simulink model "rfpsc"  (R2023b)
settings: Solver=VariableStepAuto  StartTime=0.0  StopTime=.5  RelTol=1e-3
undefined symbols (not defined in the file): f_sw, K_p, L_f, L_g, R_a, R_L, T_s, U_dc, u_gN, w_b, w_g
libraries: simulink x1
settings Model: Creator=maatt  LastModifiedBy=maatt
settings DataIOCC: ReturnWorkspaceOutputs=off

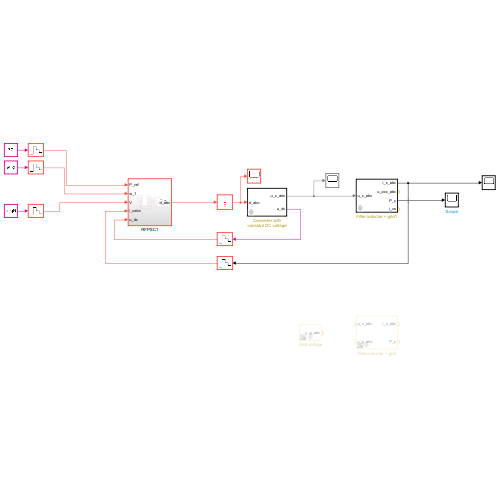
[thumbnail: Simulink's stored preview of the top-level diagram]
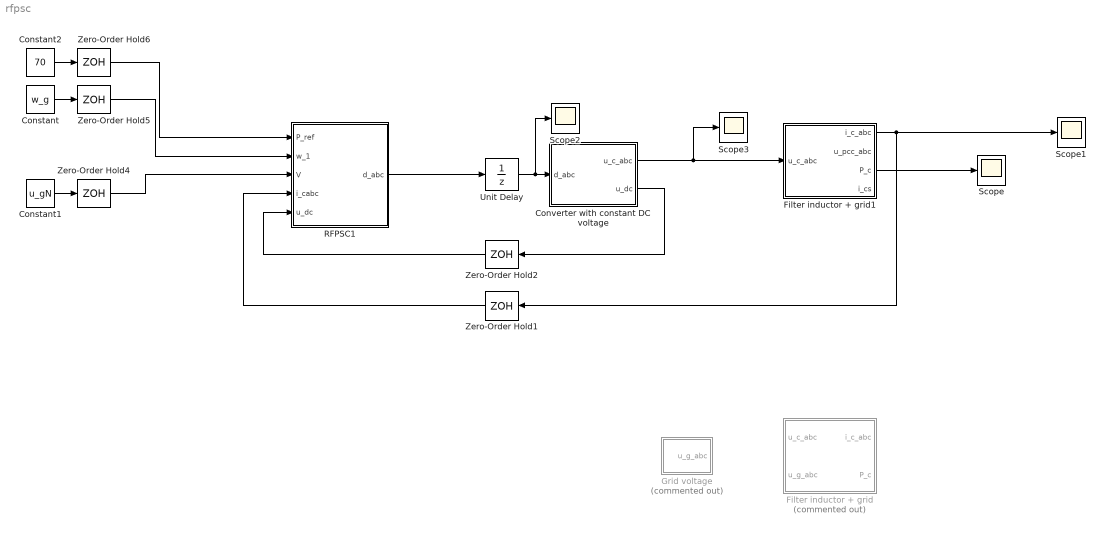
== system rfpsc ==
  Constant : Constant  Value=w_g
  Constant1 : Constant  Value=u_gN
  Constant2 : Constant  Value=70
  "Converter with constant DC voltage " : Subsystem  mask{f_sw=f_sw, u_dc=U_dc}
      mask prompts: f_sw "Switching frequency (Hz)"; u_dc "DC-bus voltage (V)"
      mask init:
      | T_s = 1/(2*f_sw);
  Filter inductor + grid : Subsystem  Commented=on  mask{L_f=L_f, L_g=L_g, R_L=R_L}
      mask prompts: L_f "Filter inductance (H)"; L_g "Grid inductance (H)"; R_L "Series resistance (ohm)"
  Filter inductor + grid1 : Subsystem  mask{L_f=L_f, L_g=L_g, R_L=R_L}
      mask prompts: L_f "Filter inductance (H)"; L_g "Grid inductance (H)"; R_L "Series resistance (ohm)"
  Grid voltage : Subsystem  Commented=on  mask{w_g=2*pi*50, U_g=24}
      mask prompts: w_g "Grid angular frequency (rad/s)"; U_g "Line-to-neutral peak voltage (V)"
  RFPSC1 : Subsystem
  Scope{,1..3} (4 alike) : Scope
  Unit Delay : UnitDelay  SampleTime=T_s  HasFrameUpgradeWarning=on
  Zero-Order Hold{1..2,4..6} (5 alike) : ZeroOrderHold  SampleTime=T_s
  wires:
  "Converter with constant DC voltage "/1(u_c_abc) -> Filter inductor + grid1/1(u_c_abc), Scope3/1
  RFPSC1/1(d_abc) -> Unit Delay/1
  "Converter with constant DC voltage "/2(u_dc) -> Zero-Order Hold2/1
  Constant/1 -> Zero-Order Hold5/1
  Constant1/1 -> Zero-Order Hold4/1
  Unit Delay/1 -> Scope2/1, "Converter with constant DC voltage "/1(d_abc)
  Zero-Order Hold1/1 -> RFPSC1/4(i_cabc)
  Zero-Order Hold4/1 -> RFPSC1/3(V)
  Zero-Order Hold5/1 -> RFPSC1/2(w_1)
  Zero-Order Hold6/1 -> RFPSC1/1(P_ref)
  Zero-Order Hold2/1 -> RFPSC1/5(u_dc)
  Constant2/1 -> Zero-Order Hold6/1
  Filter inductor + grid1/1(i_c_abc) -> Scope1/1, Zero-Order Hold1/1
  Filter inductor + grid1/3(P_c) -> Scope/1

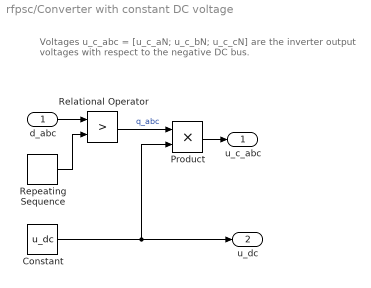
== system rfpsc/Converter with constant DC voltage  ==
  note: Voltages u_c_abc = [u_c_aN; u_c_bN; u_c_cN] are the inverter
      | output voltages with respect to the negative DC bus.
  d_abc : Inport
  Constant : Constant  Value=u_dc
  Product : Product
  Relational Operator : RelationalOperator  Operator=>  OutDataTypeStr='double'  InputSameDT=off
  Repeating Sequence : simulink/Sources/Repeating Sequence  rep_seq_t=[0 1 2]*T_s  rep_seq_y=[1 0 1]
  u_c_abc : Outport
  u_dc : Outport  Port=2
  wires:
  Repeating Sequence/1 -> Relational Operator/2
  d_abc/1 -> Relational Operator/1
  Product/1 -> u_c_abc/1
  Relational Operator/1 -> Product/1  "q_abc"
  Constant/1 -> Product/2, u_dc/1

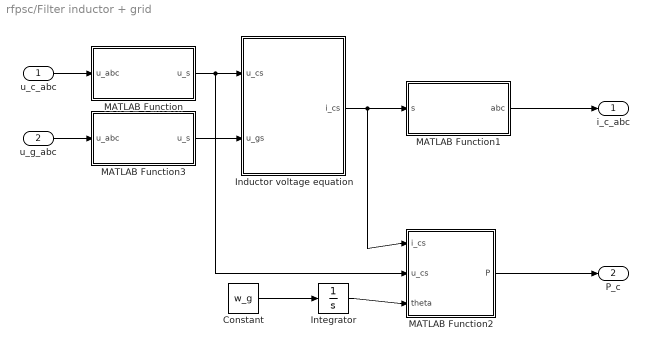
== system rfpsc/Filter inductor + grid ==
  u_c_abc : Inport
  u_g_abc : Inport  Port=2
  Constant : Constant  Value=w_g
  Inductor voltage equation : Subsystem
  Integrator : Integrator  WrapState=on
  MATLAB Function : MATLAB Function  TreatAsAtomicUnit=on
  MATLAB Function1 : MATLAB Function  TreatAsAtomicUnit=on
  MATLAB Function2 : MATLAB Function  TreatAsAtomicUnit=on
  MATLAB Function3 : MATLAB Function  TreatAsAtomicUnit=on
  i_c_abc : Outport
  P_c : Outport  Port=2
  wires:
  u_c_abc/1 -> MATLAB Function/1(u_abc)
  MATLAB Function/1(u_s) -> MATLAB Function2/2(u_cs), Inductor voltage equation/1(u_cs)
  u_g_abc/1 -> MATLAB Function3/1(u_abc)
  MATLAB Function3/1(u_s) -> Inductor voltage equation/2(u_gs)
  Inductor voltage equation/1(i_cs) -> MATLAB Function2/1(i_cs), MATLAB Function1/1(s)
  MATLAB Function1/1(abc) -> i_c_abc/1
  Constant/1 -> Integrator/1
  Integrator/1 -> MATLAB Function2/3(theta)
  MATLAB Function2/1(P) -> P_c/1

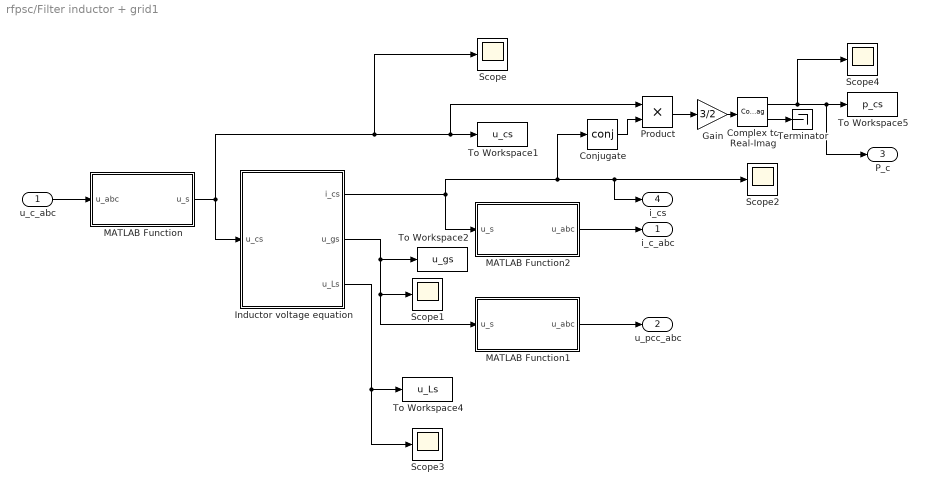
== system rfpsc/Filter inductor + grid1 ==
  u_c_abc : Inport
  Complex to Real-Imag : ComplexToRealImag
  Conjugate : Math  Operator=conj  SignedPower=on  RndMeth=Zero
  Gain : Gain  Gain=3/2
  Inductor voltage equation : Subsystem
  MATLAB Function : MATLAB Function  TreatAsAtomicUnit=on
  MATLAB Function1 : MATLAB Function  TreatAsAtomicUnit=on
  MATLAB Function2 : MATLAB Function  TreatAsAtomicUnit=on
  Product : Product
  Scope{,1..4} (5 alike) : Scope
  Terminator : Terminator
  To Workspace1 : ToWorkspace  VariableName=u_cs  SaveFormat=Timeseries
  To Workspace2 : ToWorkspace  VariableName=u_gs  SaveFormat=Timeseries
  To Workspace4 : ToWorkspace  VariableName=u_Ls  SaveFormat=Timeseries
  To Workspace5 : ToWorkspace  VariableName=p_cs  SaveFormat=Timeseries
  i_c_abc : Outport
  u_pcc_abc : Outport  Port=2
  P_c : Outport  Port=3
  i_cs : Outport  Port=4
  wires:
  u_c_abc/1 -> MATLAB Function/1(u_abc)
  Inductor voltage equation/1(i_cs) -> i_cs/1, Scope2/1, Conjugate/1, MATLAB Function2/1(u_s)
  MATLAB Function2/1(u_abc) -> i_c_abc/1
  MATLAB Function/1(u_s) -> Inductor voltage equation/1(u_cs), Scope/1, Product/1, To Workspace1/1
  Inductor voltage equation/2(u_gs) -> Scope1/1, MATLAB Function1/1(u_s), To Workspace2/1
  Inductor voltage equation/3(u_Ls) -> To Workspace4/1, Scope3/1
  MATLAB Function1/1(u_abc) -> u_pcc_abc/1
  Conjugate/1 -> Product/2
  Complex to Real-Imag/1 -> Scope4/1, P_c/1, To Workspace5/1
  Complex to Real-Imag/2 -> Terminator/1
  Product/1 -> Gain/1
  Gain/1 -> Complex to Real-Imag/1

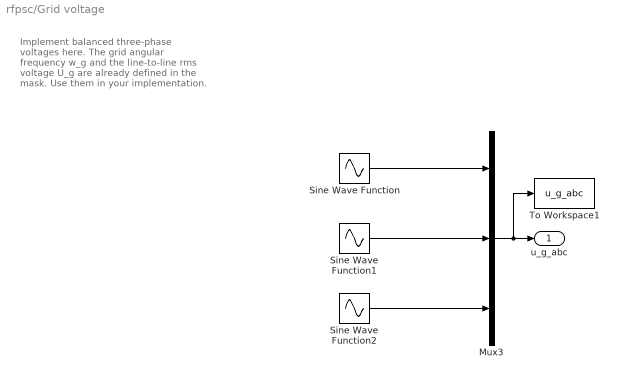
== system rfpsc/Grid voltage ==
  note: Implement balanced three-phase
      | voltages here. The grid angular
      | frequency w_g and the line-to-line rms
      | voltage U_g are already defined
      | in the mask. Use them in your
      | implementation.
  Mux3 : Mux  Inputs=3
  Sine Wave Function : Sin  Amplitude=U_g*sqrt(2/3)  Frequency=w_g
  Sine Wave Function1 : Sin  Amplitude=U_g*sqrt(2/3)  Frequency=w_g  Phase=2*pi/3
  Sine Wave Function2 : Sin  Amplitude=U_g*sqrt(2/3)  Frequency=w_g  Phase=4*pi/3
  To Workspace1 : ToWorkspace  VariableName=u_g_abc  SaveFormat=Timeseries  SampleTime=-1
  u_g_abc : Outport
  wires:
  Mux3/1 -> To Workspace1/1, u_g_abc/1
  Sine Wave Function/1 -> Mux3/1
  Sine Wave Function1/1 -> Mux3/2
  Sine Wave Function2/1 -> Mux3/3

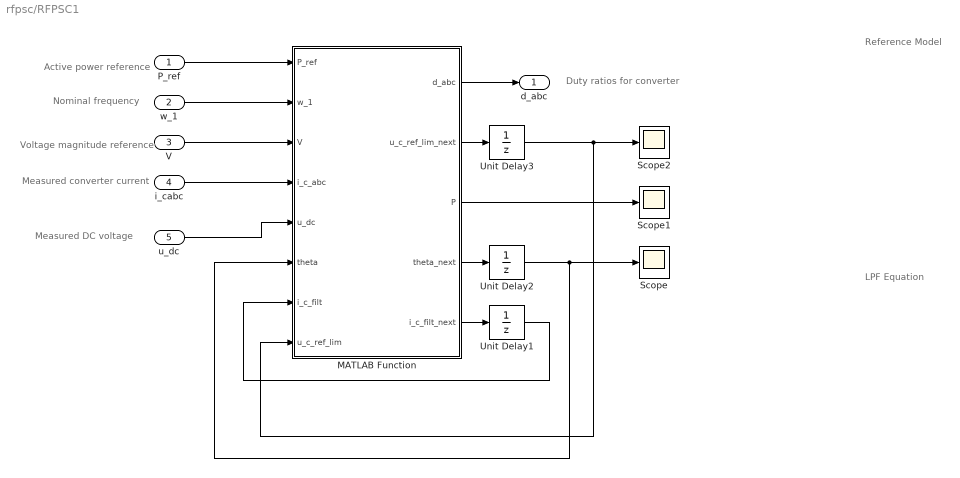
== system rfpsc/RFPSC1 ==
  note: Measured DC voltage
  note: Voltage magnitude reference
  note: Nominal frequency
  note: Measured converter current
  note: Active power reference
  note: Duty ratios for converter
  note: Reference Model
  note: LPF Equation
  P_ref : Inport
  w_1 : Inport  Port=2
  V : Inport  Port=3
  i_cabc : Inport  Port=4
  u_dc : Inport  Port=5
  MATLAB Function : MATLAB Function  TreatAsAtomicUnit=on
  Scope : Scope
  Scope1 : Scope
  Scope2 : Scope
  Unit Delay1 : UnitDelay  SampleTime=-1  HasFrameUpgradeWarning=on
  Unit Delay2 : UnitDelay  SampleTime=-1  HasFrameUpgradeWarning=on
  Unit Delay3 : UnitDelay  SampleTime=-1  HasFrameUpgradeWarning=on
  d_abc : Outport
  wires:
  P_ref/1 -> MATLAB Function/1(P_ref)
  w_1/1 -> MATLAB Function/2(w_1)
  V/1 -> MATLAB Function/3(V)
  i_cabc/1 -> MATLAB Function/4(i_c_abc)
  MATLAB Function/1(d_abc) -> d_abc/1
  MATLAB Function/5(i_c_filt_next) -> Unit Delay1/1
  Unit Delay1/1 -> MATLAB Function/7(i_c_filt)
  MATLAB Function/4(theta_next) -> Unit Delay2/1
  Unit Delay2/1 -> MATLAB Function/6(theta), Scope/1
  u_dc/1 -> MATLAB Function/5(u_dc)
  MATLAB Function/2(u_c_ref_lim_next) -> Unit Delay3/1
  MATLAB Function/3(P) -> Scope1/1
  Unit Delay3/1 -> MATLAB Function/8(u_c_ref_lim), Scope2/1

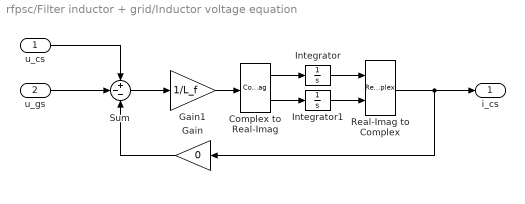
== system rfpsc/Filter inductor + grid/Inductor voltage equation ==
  u_cs : Inport
  u_gs : Inport  Port=2
  Complex to Real-Imag : ComplexToRealImag
  Gain : Gain  Gain=0
  Gain1 : Gain  Gain=1/L_f
  Integrator : Integrator
  Integrator1 : Integrator
  Real-Imag to Complex : RealImagToComplex
  Sum : Sum  Inputs=+--
  i_cs : Outport
  wires:
  Real-Imag to Complex/1 -> Gain/1, i_cs/1
  Gain/1 -> Sum/3
  Sum/1 -> Gain1/1
  u_gs/1 -> Sum/2
  Gain1/1 -> Complex to Real-Imag/1
  u_cs/1 -> Sum/1
  Integrator/1 -> Real-Imag to Complex/1
  Complex to Real-Imag/1 -> Integrator/1
  Complex to Real-Imag/2 -> Integrator1/1
  Integrator1/1 -> Real-Imag to Complex/2

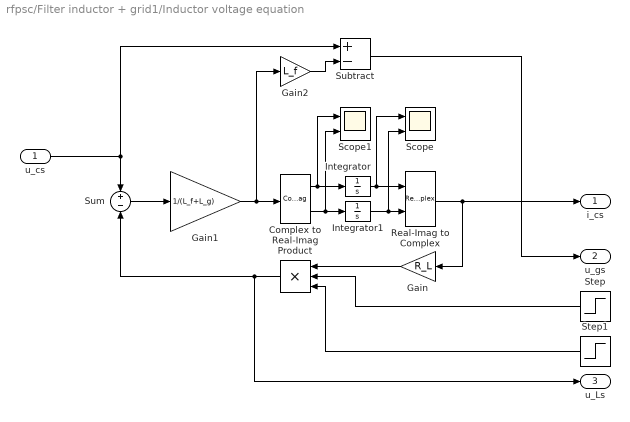
== system rfpsc/Filter inductor + grid1/Inductor voltage equation ==
  u_cs : Inport
  Complex to Real-Imag : ComplexToRealImag
  Gain : Gain  Gain=R_L
  Gain1 : Gain  Gain=1/(L_f+L_g)
  Gain2 : Gain  Gain=L_f
  Integrator : Integrator
  Integrator1 : Integrator
  Product : Product  Inputs=3
  Real-Imag to Complex : RealImagToComplex
  Scope : Scope  NumInputPorts=2
  Scope1 : Scope  NumInputPorts=2
  Step : Step  Time=0.05  Before=1  After=2  SampleTime=0
  Step1 : Step  Time=0.08  Before=1  SampleTime=0
  Subtract : Sum  Inputs=+-
  Sum : Sum  Inputs=+|-
  i_cs : Outport
  u_gs : Outport  Port=2
  u_Ls : Outport  Port=3
  wires:
  u_cs/1 -> Subtract/1, Sum/1
  Sum/1 -> Gain1/1
  Gain1/1 -> Gain2/1, Complex to Real-Imag/1
  Complex to Real-Imag/1 -> Scope1/1, Integrator/1
  Complex to Real-Imag/2 -> Scope1/2, Integrator1/1
  Integrator/1 -> Scope/1, Real-Imag to Complex/1
  Integrator1/1 -> Scope/2, Real-Imag to Complex/2
  Real-Imag to Complex/1 -> i_cs/1, Gain/1
  Gain/1 -> Product/1
  Gain2/1 -> Subtract/2
  Subtract/1 -> u_gs/1
  Step/1 -> Product/2
  Product/1 -> u_Ls/1, Sum/2
  Step1/1 -> Product/3

== matlab function rfpsc/Filter inductor + grid1/MATLAB Function2 ==
  data: u_s input size=1; u_abc output size=3
function u_abc = s2abc(u_s)

% Inverse space-vector transformation
u_abc = real([1; exp(-1j*2*pi/3); exp(-1j*4*pi/3)]*u_s);

== matlab function rfpsc/RFPSC1/MATLAB Function ==
  data: P_ref input; d_abc output; u_c_ref_lim_next output; P output; theta_next output; w_1 input; V input; i_c_abc input; u_dc input; theta input; i_c_filt input; K_p parameter; T_s parameter; R_a parameter; i_c_filt_next output; w_b parameter; u_c_ref_lim input
function [d_abc, u_c_ref_lim_next, P, theta_next, i_c_filt_next] = RFPSC(P_ref, w_1, V, i_c_abc, u_dc,...
   theta, i_c_filt, K_p, T_s, R_a, w_b, u_c_ref_lim)

% Space Vector Transformation of converter current (abcTos)
i_cs = 2/3*(i_c_abc(1) + i_c_abc(2)*exp(1j*2*pi/3) + i_c_abc(3)*exp(1j*4*pi/3));

% Coordinate transformation of converter current
i_c = i_cs*exp(-1j*theta);

% Active power calculation
P = 3/2*real(u_c_ref_lim*conj(i_c));

% Equation for grid angular frequency
w_g = (P_ref - P)*K_p + w_1;

% Update (integrate) the grid voltage angle
theta_next = theta + T_s * w_g; % Discrete time compensation
while(theta_next > pi)
    theta_next = theta_next - 2*pi;
end
while(theta_next < -pi)
    theta_next = theta_next + 2*pi;
end

% Extracting the real and imaginary values of the complex converter current
i_c_imag = imag(i_c);

% Applying lowpass filter equation to imaginary part of the
% converter current and forming reference current based on power reference
i_c_filt_next =  i_c_filt*(1 - w_b*T_s) + i_c_imag*(w_b*T_s);
i_ref = P_ref/V + 1j*i_c_filt_next;

% Equation for reference voltage
u_c = V + (i_ref-i_c) * R_a;

% Inverse coordinate transformation
u_cs_ref = u_c*exp(1j*(theta + 1.5 * T_s * w_1));


%% Symmetrical suboscillation PWM
% Components of the voltage space vector
u_c_alpha_ref = real(u_cs_ref);
u_c_beta_ref  = imag(u_cs_ref);

% Phase-voltage references
u_ca_ref = u_c_alpha_ref;
u_cb_ref = .5*(-u_c_alpha_ref + sqrt(3)*u_c_beta_ref);
u_cc_ref = .5*(-u_c_alpha_ref - sqrt(3)*u_c_beta_ref);

% Vector of phase-voltage references
u_c_abc_ref = [u_ca_ref; u_cb_ref; u_cc_ref];

% Symmetrization of the references by adding the zero-sequence voltage
u0 = .5*(max(u_c_abc_ref) + min(u_c_abc_ref));
u_c_abc_ref = u_c_abc_ref - u0;

% Clipping of the reference voltages such that no phase error is caused. 
% If all phase voltage reference are realizable (below u_dc/2), m = 1 holds.
m = max([2*u_c_abc_ref/u_dc; 1]);
u_c_abc_ref = u_c_abc_ref/m;

% Duty cycles, which can be directly used for triangle comparison, 
% if the triangle wave varies between 0...1
d_abc = .5 + u_c_abc_ref/u_dc;
% 
% % Realized voltage vector is calculated from the clamped duty ratios.
% % If the PWM does not saturate, u_c_ref_lim = u_c_ref holds. The realized
% % voltage vector is needed, e.g., for the current-controller antiwindup.
u_cs_ref_lim = 2/3*(d_abc(1) + d_abc(2)*exp(1j*2*pi/3) ...
     + d_abc(3)*exp(1j*4*pi/3))*u_dc;
% % In estimated rotor flux coordinates
u_c_ref_lim_next = exp(-1j*(theta + 1.5 * T_s * w_1))*u_cs_ref_lim;

== matlab function rfpsc/Filter inductor + grid/MATLAB Function3 ==
  data: u_abc input size=3; u_s output size=1
function u_s = abc2s(u_abc)

% Space-vector transformation
u_s = 2/3*(u_abc(1) + u_abc(2)*exp(1j*2*pi/3) + u_abc(3)*exp(1j*4*pi/3));

== matlab function rfpsc/Filter inductor + grid/MATLAB Function1 ==
  data: s input size=1; abc output size=3
function abc = s2abc(s)

% Inverse space-vector transformation
abc = real([1; exp(-1j*2*pi/3); exp(-1j*4*pi/3)]*s);

== matlab function rfpsc/Filter inductor + grid/MATLAB Function2 ==
  data: i_cs input; P output; u_cs input; theta input
function P = fcn(i_cs, u_cs, theta)

% Coordinate transformation
i_c = i_cs*exp(-1j*theta);
u_c = u_cs*exp(-1j*theta);

% Active power calculation
P = 3/2*real(u_c*conj(i_c));

== matlab function rfpsc/Filter inductor + grid/MATLAB Function ==
  data: u_abc input size=3; u_s output size=1
function u_s = abc2s(u_abc)

% Space-vector transformation
u_s = 2/3*(u_abc(1) + u_abc(2)*exp(1j*2*pi/3) + u_abc(3)*exp(1j*4*pi/3));

== matlab function rfpsc/Filter inductor + grid1/MATLAB Function ==
  data: u_abc input size=3; u_s output size=1
function u_s = abc2s(u_abc)

% Space-vector transformation
u_s = 2/3*(u_abc(1) + u_abc(2)*exp(1j*2*pi/3) + u_abc(3)*exp(1j*4*pi/3));

== matlab function rfpsc/Filter inductor + grid1/MATLAB Function1 ==
  data: u_s input size=1; u_abc output size=3
function u_abc = s2abc(u_s)

% Inverse space-vector transformation
u_abc = real([1; exp(-1j*2*pi/3); exp(-1j*4*pi/3)]*u_s);
